simulink model "PLL"  (R2022b)
settings: Solver=ode23t  StartTime=0.0  StopTime=0.08  RelTol=1e-3
libraries: spsSeriesRLCBranchLib x2, spsVoltageMeasurementLib x2, spsACVoltageSourceLib x1, simulink x1, spsCurrentMeasurementLib x1, dspsigops x1, sps_lib x1
settings Model: Creator=HP  LastModifiedBy=dell

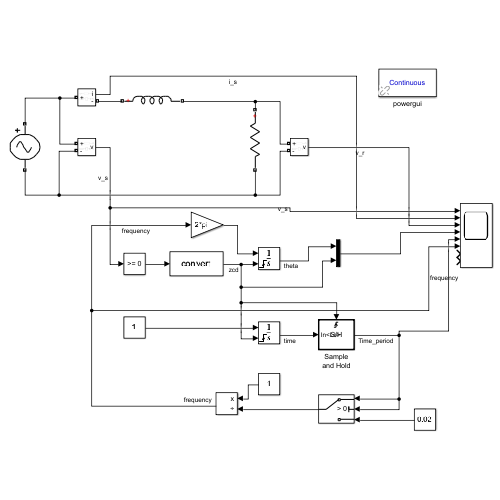
[thumbnail: Simulink's stored preview of the top-level diagram]
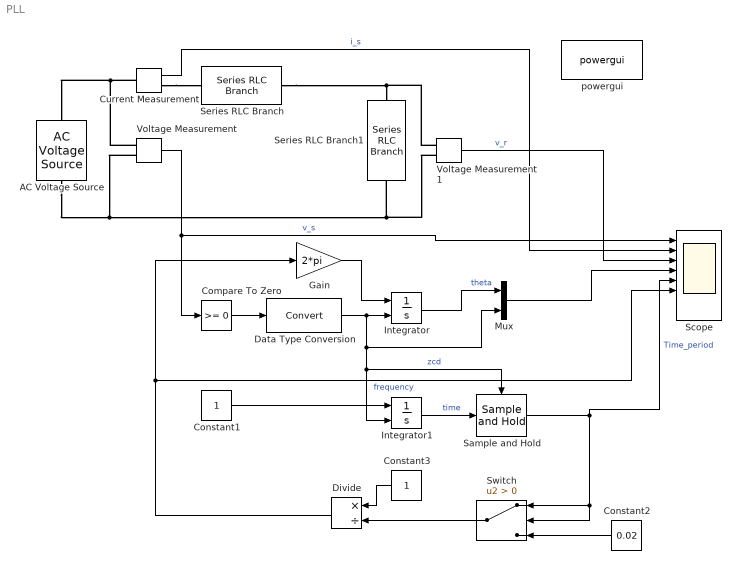
== system PLL ==
  AC Voltage Source : spsACVoltageSourceLib/AC Voltage Source  Amplitude=230*sqrt(2)  Phase=0  Frequency=30  SampleTime=0  Measurements=None  BusType=swing  Pref=10e3  Qref=0  Qmin=-inf  Qmax=+inf
  Compare To Zero : simulink/Logic and Bit Operations/Compare To Zero  relop=>=  OutDataTypeStr=boolean
  Constant1 : Constant
  Constant2 : Constant  Value=0.02
  Constant3 : Constant
  Current Measurement : spsCurrentMeasurementLib/Current Measurement  PhasorSimulation=off  OutputType=Complex  PSBequivalent=0
  Data Type Conversion : DataTypeConversion  SaturateOnIntegerOverflow=off  RndMeth=Floor
  Divide : Product  Inputs=*/
  Gain : Gain  Gain=2*pi
  Integrator : Integrator  ExternalReset=rising
  Integrator1 : Integrator  ExternalReset=rising
  Mux : Mux  Inputs=2
  Sample and Hold : dspsigops/Sample and Hold  trig=Rising edge  initCond=0  latchinput=on
  Scope : Scope  NumInputPorts=8
  Series RLC Branch : spsSeriesRLCBranchLib/Series RLC Branch  LConnTagsString=__new0  RConnTagsString=__new0  BranchType=L  Resistance=1  Inductance=12.7e-3  SetiL0=off  InitialCurrent=0  Capacitance=1e-6  Setx0=off  InitialVoltage=0  Measurements=None
  Series RLC Branch1 : spsSeriesRLCBranchLib/Series RLC Branch  LConnTagsString=__new0  RConnTagsString=__new0  BranchType=R  Resistance=10  Inductance=12.7e-3  SetiL0=off  InitialCurrent=0  Capacitance=1e-6  Setx0=off  InitialVoltage=0  Measurements=None
  Switch : Switch  Criteria=u2 > Threshold  SaturateOnIntegerOverflow=off  InputSameDT=off
  Voltage Measurement : spsVoltageMeasurementLib/Voltage Measurement  PhasorSimulation=off  OutputType=Complex  PSBequivalent=0
  Voltage Measurement1 : spsVoltageMeasurementLib/Voltage Measurement  PhasorSimulation=off  OutputType=Complex  PSBequivalent=0
  powergui : sps_lib/powergui  Priority=1  SimulationMode=Continuous  SampleTime=50e-6  frequency=60  Iterations=50  frequencyindice=30  Pbase=100e6  ErrMax=1e-4  UnitsV=kV  UnitsW=MW  buscounter=0  FunctionMessages=off  echomessages=off  EnableUseOfTLC=off  CurrentSourceSwitches=off  DisableSnubberDevices=off  DisableRonSwitches=off  DisableVfSwitches=off  DisplayEquations=off  AutomaticDiscreteSolvers=off  SolverType=Tustin/Backward Euler (TBE)  Interpol=off  ExternalGateDelay=off  methode=off  Ts=100  x0status=blocks  SPID=on  SwTol=0  HookPort=off  NonlinearTolerance=1e-4  nMaxIteration=100  ContinueOnMaxIteration=off  RestoreLinks=warning  ResistiveCurrentMeasurement=off  Frange=[0:2:500]  Ylog=off  Xlog=on  ShowGrid=off  save=off  variable=ZData  structure=0  ZoomFFT=off  StartTime=0.0  cycles=1  DisplayStyle=1  fundamental=60  FreqAxis=off  MaxFrequency=1000  frequencyindicesteady=1  RmsSteady=1  display=off
  wires:
  Voltage Measurement/1 -> Scope/1, Compare To Zero/1  "v_s"
  Compare To Zero/1 -> Data Type Conversion/1
  Data Type Conversion/1 -> Sample and Hold/Trigger, Integrator1/2, Mux/2, Integrator/2  "zcd"
  Gain/1 -> Integrator/1
  Current Measurement/1 -> Scope/2  "i_s"
  Voltage Measurement1/1 -> Scope/3  "v_r"
  Mux/1 -> Scope/4
  Integrator/1 -> Mux/1  "theta"
  Constant1/1 -> Integrator1/1
  Integrator1/1 -> Sample and Hold/1  "time"
  Sample and Hold/1 -> Switch/2, Switch/1, Scope/5  "Time_period"
  Switch/1 -> Divide/2
  Constant2/1 -> Switch/3
  Constant3/1 -> Divide/1
  Divide/1 -> Gain/1, Scope/6  "frequency"
  connections:
  AC Voltage Source/LConn1 -- Voltage Measurement1/LConn2 -- Series RLC Branch1/RConn1 -- Voltage Measurement/LConn2
  Series RLC Branch/RConn1 -- Voltage Measurement1/LConn1 -- Series RLC Branch1/LConn1
  Current Measurement/RConn1 -- Series RLC Branch/LConn1
  Current Measurement/LConn1 -- Voltage Measurement/LConn1 -- AC Voltage Source/RConn1
